simulink model "fix_point"  (R2022a)
settings: Solver=VariableStepAuto  StartTime=0.0  StopTime=10.0  RelTol=1e-3
settings Model: Creator=User  LastModifiedBy=User

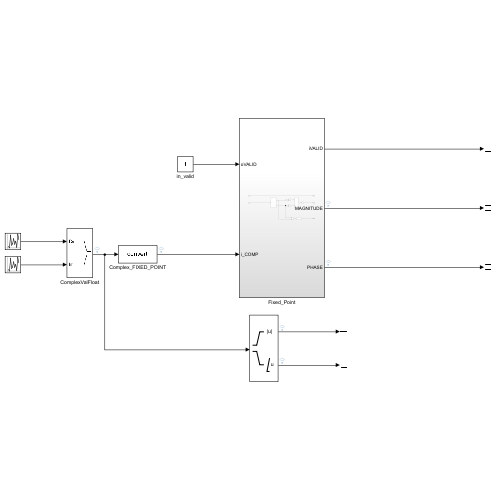
[thumbnail: Simulink's stored preview of the top-level diagram]
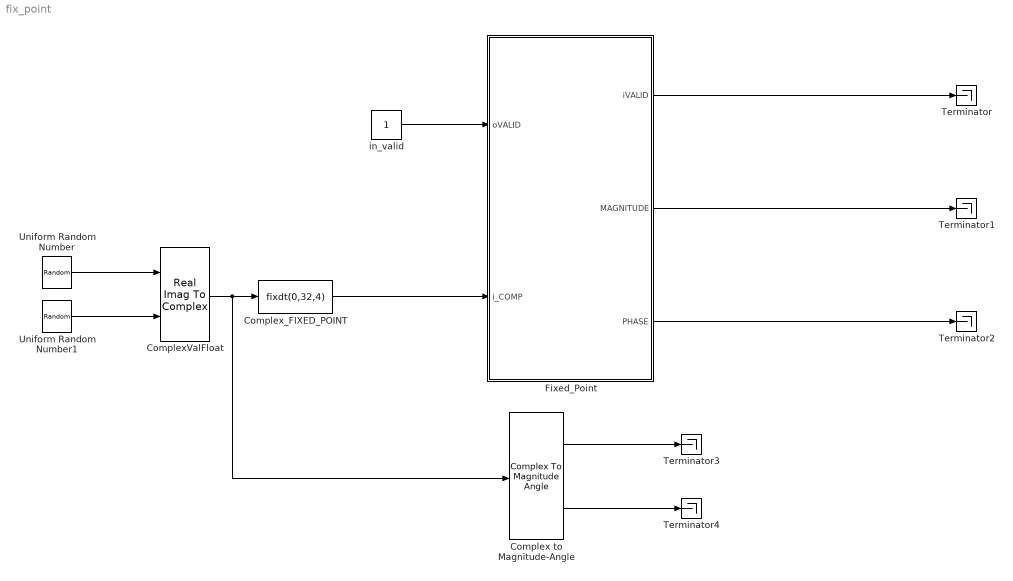
== system fix_point ==
  Complex to Magnitude-Angle : ComplexToMagnitudeAngle
  ComplexValFloat : RealImagToComplex
  Complex_FIXED_POINT : DataTypeConversion  OutDataTypeStr=fixdt(0,32,4)  RndMeth=Round  SaturateOnIntegerOverflow=off
  Fixed_Point : Subsystem
  Terminator{,1..4} (5 alike) : Terminator
  Uniform Random Number : UniformRandomNumber  Minimum=0  Maximum=2 ^(28) - 1  Seed=28  SampleTime=1
  Uniform Random Number1 : UniformRandomNumber  Minimum=0  Maximum=2 ^(28) - 1  Seed=28  SampleTime=1
  in_valid : Constant  OutDataTypeStr=boolean  SampleTime=1
  wires:
  Complex to Magnitude-Angle/2 -> Terminator4/1
  Fixed_Point/1(iVALID) -> Terminator/1
  Uniform Random Number/1 -> ComplexValFloat/1
  Uniform Random Number1/1 -> ComplexValFloat/2
  Fixed_Point/2(MAGNITUDE) -> Terminator1/1
  ComplexValFloat/1 -> Complex to Magnitude-Angle/1, Complex_FIXED_POINT/1
  Complex_FIXED_POINT/1 -> Fixed_Point/2(i_COMP)
  Complex to Magnitude-Angle/1 -> Terminator3/1
  Fixed_Point/3(PHASE) -> Terminator2/1
  in_valid/1 -> Fixed_Point/1(oVALID)

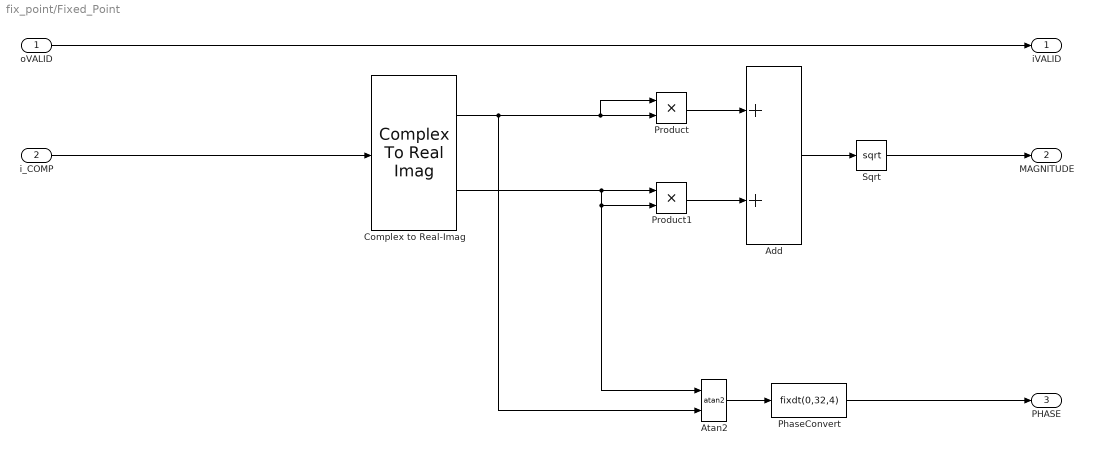
== system fix_point/Fixed_Point ==
  oVALID : Inport  OutDataTypeStr=boolean
  i_COMP : Inport  Port=2
  Add : Sum
  Atan2 : Trigonometry  Operator=atan2  ApproximationMethod=CORDIC
  Complex to Real-Imag : ComplexToRealImag
  PhaseConvert : DataTypeConversion  OutDataTypeStr=fixdt(0,32,4)  RndMeth=Round  SaturateOnIntegerOverflow=off
  Product : Product
  Product1 : Product
  Sqrt : Sqrt  OutDataTypeStr=fixdt(1,33,4)
  iVALID : Outport
  MAGNITUDE : Outport  Port=2
  PHASE : Outport  Port=3
  wires:
  Add/1 -> Sqrt/1
  Product/1 -> Add/1
  Sqrt/1 -> MAGNITUDE/1
  Product1/1 -> Add/2
  Atan2/1 -> PhaseConvert/1
  i_COMP/1 -> Complex to Real-Imag/1
  oVALID/1 -> iVALID/1
  PhaseConvert/1 -> PHASE/1
  Complex to Real-Imag/2 -> Atan2/1, Product1/2, Product1/1
  Complex to Real-Imag/1 -> Product/1, Product/2, Atan2/2
